simulink model "integrator_estimator"  (R2017b)
settings: Solver=FixedStepDiscrete  StartTime=0.0  StopTime=T  FixedStep=0.01  RelTol=1e-3
values from neighbouring files (symbols this model uses):
  rollGrad = 5*(pi/180)    (= 0.0872664625997)    [Init_for_washout_filter.m]
undefined symbols (not defined in the file or in its folder): DiscIntNeverNeededParam
settings Model: Creator=gandh  LastModifiedBy=gandh

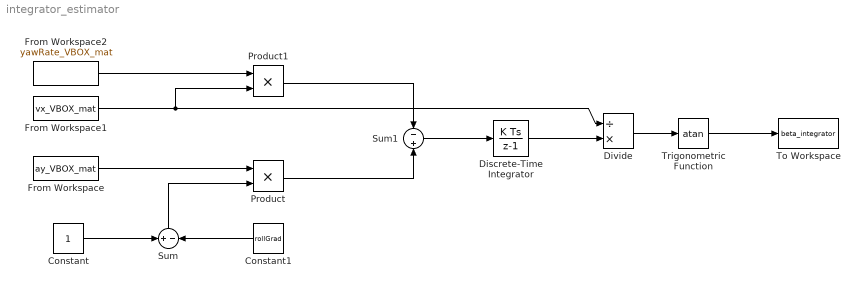
== system integrator_estimator ==
  Constant : Constant
  Constant1 : Constant  Value=rollGrad
  Discrete-Time Integrator : DiscreteIntegrator  InitialConditionSetting=State (most efficient)  SampleTime=-1  ICPrevOutput=DiscIntNeverNeededParam  ICPrevScaledInput=DiscIntNeverNeededParam
  Divide : Product  Inputs=/*
  From Workspace : FromWorkspace  VariableName=ay_VBOX_mat  SampleTime=0
  From Workspace1 : FromWorkspace  VariableName=vx_VBOX_mat  SampleTime=0
  From Workspace2 : FromWorkspace  VariableName=yawRate_VBOX_mat  SampleTime=0
  Product : Product
  Product1 : Product
  Sum : Sum  Inputs=+-
  Sum1 : Sum  Inputs=-+
  To Workspace : ToWorkspace  VariableName=beta_integrator  SaveFormat=Timeseries  SampleTime=-1
  Trigonometric Function : Trigonometry  Operator=atan
  wires:
  Constant/1 -> Sum/1
  Constant1/1 -> Sum/2
  From Workspace/1 -> Product/1
  Sum/1 -> Product/2
  From Workspace2/1 -> Product1/1
  From Workspace1/1 -> Divide/1, Product1/2
  Product/1 -> Sum1/2
  Product1/1 -> Sum1/1
  Sum1/1 -> Discrete-Time Integrator/1
  Divide/1 -> Trigonometric Function/1
  Trigonometric Function/1 -> To Workspace/1
  Discrete-Time Integrator/1 -> Divide/2
